simulink model "batery_model"  (R2017b)
settings: Solver=VariableStepAuto  StartTime=0.0  StopTime=sim_time  RelTol=1e-3
values from neighbouring files (symbols this model uses):
  Cn = 2.3*3600    (= 8280)    [Battery_parameter.m]
  I = 2.3    [Battery_parameter.m]
  ocv = data(:,2)    [Battery_parameter.m]
  r_charge = data(:,3)    [Battery_parameter.m]
  r_discharge = data(:,4)    [Battery_parameter.m]
  soc = data(:,1)    [Battery_parameter.m]
settings Model: Creator=Tapas  LastModifiedBy=Tapas

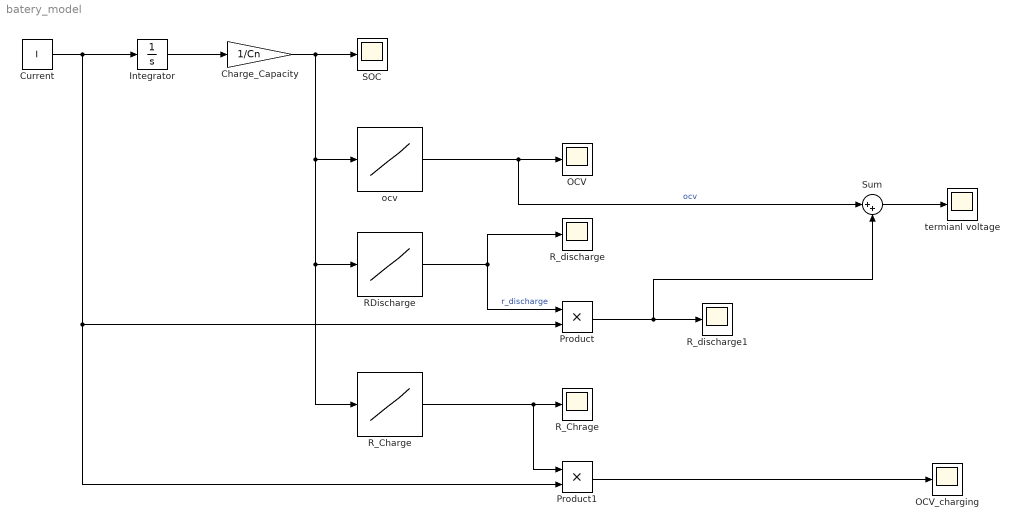
== system batery_model ==
  Charge_Capacity : Gain  Gain=1/Cn
  Current : Constant  Value=I
  Integrator : Integrator
  OCV : Scope
  OCV_charging : Scope
  Product : Product
  Product1 : Product
  RDischarge : Lookup_n-D  NumberOfTableDimensions=1  BreakpointsForDimension1=soc  Table=r_discharge  InternalRulePriority=Speed  RndMeth=Simplest  InputSameDT=on
  R_Charge : Lookup_n-D  NumberOfTableDimensions=1  BreakpointsForDimension1=soc  Table=r_charge  InternalRulePriority=Speed  RndMeth=Simplest  InputSameDT=on
  R_Chrage : Scope
  R_discharge : Scope
  R_discharge1 : Scope
  SOC : Scope
  Sum : Sum  Inputs=|++
  ocv : Lookup_n-D  NumberOfTableDimensions=1  BreakpointsForDimension1=soc  Table=ocv  InternalRulePriority=Speed  RndMeth=Simplest  InputSameDT=on
  termianl voltage : Scope
  wires:
  Current/1 -> Product/2, Product1/2, Integrator/1
  Integrator/1 -> Charge_Capacity/1
  Charge_Capacity/1 -> ocv/1, R_Charge/1, RDischarge/1, SOC/1
  RDischarge/1 -> R_discharge/1, Product/1  "r_discharge"
  ocv/1 -> Sum/1, OCV/1  "ocv"
  Product/1 -> Sum/2, R_discharge1/1
  Sum/1 -> termianl voltage/1
  R_Charge/1 -> Product1/1, R_Chrage/1
  Product1/1 -> OCV_charging/1
